simulink model "srf_pll_test"  (R2026a)
settings: Solver=FixedStepDiscrete  StopTime=0.3  FixedStep=1e-5
model workspace (MATLAB code in the model file):
  | % SRF-PLL test parameters
  | Ts_pll = 1e-4;            % s   PLL rate (= inverter control rate ip.Ts_ctrl)
  | f0 = 50;                  % Hz  nominal grid frequency
  | Vpk = 400*sqrt(2/3);      % V   phase peak for 400 V line-line
  | % PLL gains are set on the SRF_PLL block mask
  | % source: [Vpk f0  t_fstep df_Hz  t_phjump dphi_deg  t_sag sag_pu  h5_pu h7_pu]
  | srcp = [Vpk f0  inf 0  inf 0  inf 1  0 0];
libraries: srfPllLib x1
settings Model: Creator=aqiba  LastModifiedBy=aqiba

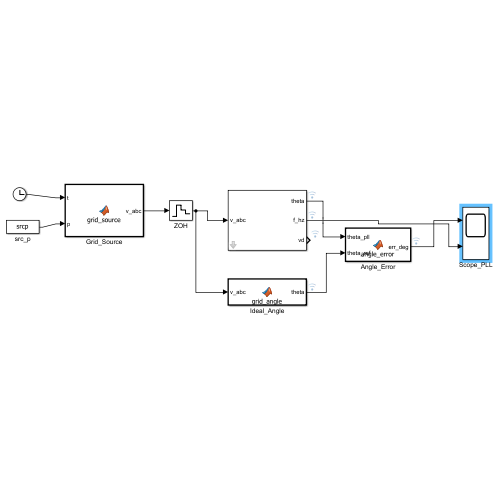
[thumbnail: Simulink's stored preview of the top-level diagram]
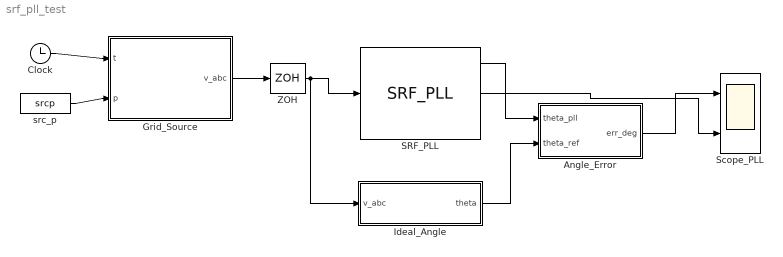
== system srf_pll_test ==
  Angle_Error : MATLAB Function  TreatAsAtomicUnit=on
  Clock : Clock
  Grid_Source : MATLAB Function  TreatAsAtomicUnit=on
  Ideal_Angle : MATLAB Function  TreatAsAtomicUnit=on
  SRF_PLL : srfPllLib/SRF_PLL  Ts=Ts_pll  f0=50  fbw=25  zeta=0.707
  Scope_PLL : Scope  NumInputPorts=2
      settings: ActiveDisplayYMinimum=-7.7039153565988752  ActiveDisplayYMaximum=56.522690733939932
  ZOH : ZeroOrderHold  SampleTime=Ts_pll
  src_p : Constant  Value=srcp
  wires:
  Clock/1 -> Grid_Source/1(t)
  src_p/1 -> Grid_Source/2(p)
  Grid_Source/1(v_abc) -> ZOH/1
  ZOH/1 -> SRF_PLL/1, Ideal_Angle/1(v_abc)
  SRF_PLL/1 -> Angle_Error/1(theta_pll)
  Ideal_Angle/1(theta) -> Angle_Error/2(theta_ref)
  Angle_Error/1(err_deg) -> Scope_PLL/1
  SRF_PLL/2 -> Scope_PLL/2

== matlab function srf_pll_test/Ideal_Angle ==
  data: v_abc input; theta output
function theta = grid_angle(v_abc)
% Reference: same as GridAngle_ideal in invPlantSw (no loop, no filter).
v_al = (2/3)*(v_abc(1) - 0.5*v_abc(2) - 0.5*v_abc(3));
v_be = (2/3)*(sqrt(3)/2)*(v_abc(2) - v_abc(3));
theta = atan2(v_be, v_al);

== matlab function srf_pll_test/Angle_Error ==
  data: theta_pll input; err_deg output; theta_ref input
function err_deg = angle_error(theta_pll, theta_ref)
% Wrapped angle difference, degrees.
err_deg = (mod(theta_pll - theta_ref + pi, 2*pi) - pi)*180/pi;

== matlab function srf_pll_test/Grid_Source ==
  data: t input; v_abc output; p input
function v_abc = grid_source(t, p)
% Three-phase test grid: p = [Vpk f0 t_fstep df t_phjump dphi_deg t_sag sag_pu h5 h7]
V = p(1); th = 2*pi*p(2)*t;
if t >= p(3), th = th + 2*pi*p(4)*(t - p(3)); end   % frequency step
if t >= p(5), th = th + p(6)*pi/180; end            % phase jump
if t >= p(7), V = V*p(8); end                       % voltage sag
a = [0; -2*pi/3; 2*pi/3];
v_abc = V*cos(th + a) + V*p(9)*cos(5*(th + a)) + V*p(10)*cos(7*(th + a));
